simulink model "rocket_lab"  (R2018b)
settings: Solver=FixedStepAuto  StartTime=0.0  StopTime=inf  FixedStep=0.05  RelTol=1e-3  EnableMultiTasking=on
libraries: arduinolib x4, simulink x1
settings Model: ExtModeTrigDuration=2  Creator=jome3  LastModifiedBy=jome3
settings OptimizationCC: EnhancedBackFolding=on  PassReuseOutputArgsAs=Individual arguments  MaxStackSize=64  OptimizeBlockOrder=speed  DifferentSizesBufferReuse=on  OptimizationCustomize=off
settings DebuggingCC: ParameterTunabilityLossMsg=error
settings HardwareCC: ProdBitPerPointer=32  ProdBitPerSizeT=32  ProdBitPerPtrDiffT=32  ProdLargestAtomicInteger=Long  ProdLargestAtomicFloat=Double  ProdWordSize=32  ProdHWDeviceType=ARM Compatible->ARM Cortex
settings SFSimCC: MATLABDynamicMemAlloc=off
settings RTWCC: SystemTargetFile=ert.tlc  HardwareBoard=Arduino Due  TemplateMakefile=ert_default_tmf  GenerateReport=on  Toolchain=Arduino ARM  BuildConfiguration=Faster Runs  IncludeHyperlinkInReport=on  LaunchReport=on  GenerateTraceInfo=on  GenerateTraceReport=on  GenerateTraceReportSl=on  GenerateTraceReportSf=on  GenerateTraceReportEml=on
settings CodeAppCC: ForceParamTrailComments=on  IgnoreCustomStorageClasses=off  OperatorAnnotations=on  SimulinkDataObjDesc=on  SFDataObjDesc=on  InsertBlockDesc=on
settings ERTTargetCC: SupportContinuousTime=on  SupportVariableSizeSignals=on

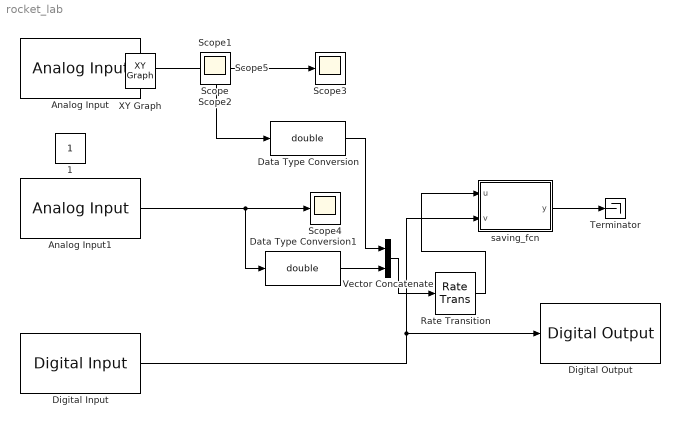
== system rocket_lab ==
  Analog Input : arduinolib/Analog Input  pinNumber=4  ReadResultsOnly=off  ConversionTriggerSource=Software  ExternalTriggerType=uint32(0)  OutputDataType=uint16  EnableConversionCompleteNotify=off  EnableOuputStatus=off  SampleTime=1  blockPlatform=arduino
  Analog Input1 : arduinolib/Analog Input  pinNumber=6  ReadResultsOnly=off  ConversionTriggerSource=Software  ExternalTriggerType=uint32(0)  OutputDataType=uint16  EnableConversionCompleteNotify=off  EnableOuputStatus=off  SampleTime=1  blockPlatform=arduino
  Data Type Conversion : DataTypeConversion  OutDataTypeStr=double
  Data Type Conversion1 : DataTypeConversion  OutDataTypeStr=double
  Digital Input : arduinolib/Digital Input  pinNumber=8  sampleTime=0.1  blockPlatform=arduino
      settings: SourceProductName=Simulink Support Package for Arduino Hardware
  Digital Output : arduinolib/Digital Output  pinNumber=9  blockPlatform=arduino
  Rate Transition : RateTransition
  Scope{,1..5} (6 alike) : Scope
  Terminator : Terminator
  Vector Concatenate : Concatenate
  "saving_fcn " : MATLAB Function  TreatAsAtomicUnit=on
  1 : Constant  IOType=siggen
  XY Graph : simulink/Sinks/XY Graph  IOType=viewer  xmin=-1  xmax=1  ymin=-1  ymax=1  st=-1
  wires:
  Analog Input/1 -> Data Type Conversion/1, Scope3/1
  Analog Input1/1 -> Data Type Conversion1/1, Scope4/1
  "saving_fcn "/1(y) -> Terminator/1
  Data Type Conversion1/1 -> Vector Concatenate/2
  Data Type Conversion/1 -> Vector Concatenate/1
  Digital Input/1 -> Digital Output/1, "saving_fcn "/2(v)
  Vector Concatenate/1 -> Rate Transition/1
  Rate Transition/1 -> "saving_fcn "/1(u)

== matlab function rocket_lab/saving_fcn  ==
  data: u input; y output; v input
function y = fcn(u, v)

if v == 1
    fname = 'text.txt';
    fid = fopen(fname, 'a+');
    fwrite(fid, u, 'double');
    fclose(fid);
    fprintf('%5.2f\n', u(1));
end

y = 1;

end
